simulink model "gravity"  (Simulink 6.1)
settings: Solver=ode45  StartTime=0.0  StopTime=10  MaxStep=2  RelTol=1e-3
libraries: Accessories_lib x1
settings Model: Creator=kkje01  LastModifiedBy=Dan T  ExtModeAutoUpdateStatusClock=off
settings DataIOCC: LimitDataPoints=off  SignalLoggingName=sigsOut
settings OptimizationCC: InlineInvariantSignals=off
settings HardwareCC: TargetUnknown=on
settings CodeAppCC: IgnoreCustomStorageClasses=off

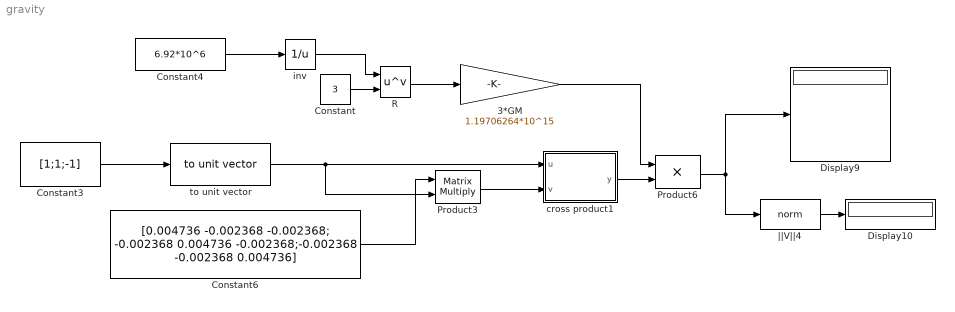
== system gravity ==
  3*GM : Gain  Gain=1.19706264*10^15  SaturateOnIntegerOverflow=on
  Constant : Constant  Value=3
  Constant3 : Constant  Value=[1;1;-1]
  Constant4 : Constant  Value=6.92*10^6
  Constant6 : Constant  Value=[0.004736 -0.002368 -0.002368; -0.002368 0.004736 -0.002368;-0.002368 -0.002368 0.004736]
  Display10 : Display
  Display9 : Display
  Product3 : Product  Multiplication=Matrix(*)  SaturateOnIntegerOverflow=on
  Product6 : Product  SaturateOnIntegerOverflow=on
  R : Math  Operator=pow  SaturateOnIntegerOverflow=on
  cross product1 : Stateflow chart
  inv : Math  Operator=reciprocal  SaturateOnIntegerOverflow=on
  to unit vector : Accessories_lib/Math utilities/Vector operations/to unit vector
  ||V||4 : MATLABFcn  MATLABFcn=norm
  wires:
  R/1 -> 3*GM/1
  inv/1 -> R/1
  Constant/1 -> R/2
  to unit vector/1 -> cross product1/1(u), Product3/2
  Product3/1 -> cross product1/2(v)
  Product6/1 -> Display9/1, ||V||4/1
  3*GM/1 -> Product6/1
  cross product1/1(y) -> Product6/2
  Constant4/1 -> inv/1
  Constant3/1 -> to unit vector/1
  Constant6/1 -> Product3/1
  ||V||4/1 -> Display10/1

== matlab function cross product1 ==
  data: u input inherited; y output inherited; v input inherited
function y = crossproduct(u,v)
% This block supports an embeddable subset of the MATLAB language.
% See the help menu for details. 

y = [u(2)*v(3)-u(3)*v(2);u(3)*v(1)-u(1)*v(3);u(1)*v(2)-u(2)*v(1)];
